simulink model "Ass3_2_2"  (R2018b)
settings: Solver=VariableStepAuto  StartTime=0.0  StopTime=40.0  RelTol=1e-3
values from neighbouring files (symbols this model uses):
  D = [X(3),0,c_0]    [Adaptive3.m]
undefined symbols (not defined in the file or in its folder): sys_m, sys_p
libraries: cstblocks x2
settings Model: Creator=bigfoot  LastModifiedBy=bigfoot

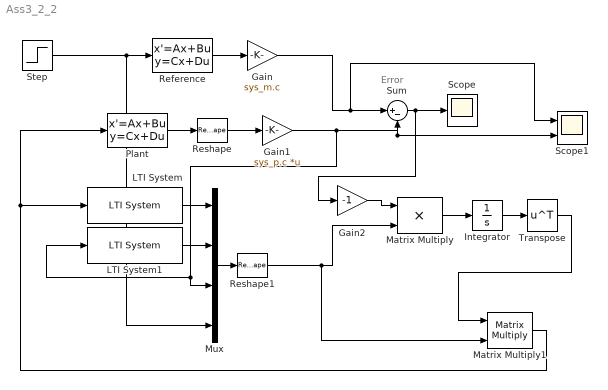
== system Ass3_2_2 ==
  note: Error
  Gain : Gain  Gain=sys_m.c
  Gain1 : Gain  Gain=sys_p.c  Multiplication=Matrix(K*u)
  Gain2 : Gain  Gain=-1
  Integrator : Integrator
  LTI System : cstblocks/LTI System  sys=tf(1,[1 1])  IC=[]
  LTI System1 : cstblocks/LTI System  sys=tf(1,[1 1])  IC=[]
  Matrix Multiply : Product
  Matrix Multiply1 : Product  Multiplication=Matrix(*)
  Mux : Mux
  Plant : StateSpace  A=sys_p.a  B=sys_p.b  C=eye(2)  D=[0;0]  InitialCondition=0
  Reference : StateSpace  A=sys_m.a  B=sys_m.b  C=eye(1)  D=[0]  InitialCondition=0
  Reshape : Reshape  OutputDimensionality=Column vector (2-D)
  Reshape1 : Reshape  OutputDimensionality=Column vector (2-D)
  Scope : Scope
  Scope1 : Scope  NumInputPorts=2
  Step : Step  SampleTime=0
  Sum : Sum  Inputs=|+-
  Transpose : Math  Operator=transpose  SaturateOnIntegerOverflow=on
  wires:
  Sum/1 -> Gain2/1, Scope/1
  Gain/1 -> Scope1/1, Sum/1
  Reference/1 -> Gain/1
  Gain1/1 -> LTI System1/1, Mux/3, Scope1/2, Sum/2
  Plant/1 -> Reshape/1
  Reshape/1 -> Gain1/1
  Step/1 -> Mux/4, Reference/1
  LTI System/1 -> Mux/1
  LTI System1/1 -> Mux/2
  Mux/1 -> Reshape1/1
  Gain2/1 -> Matrix Multiply/1
  Reshape1/1 -> Matrix Multiply1/2, Matrix Multiply/2
  Matrix Multiply/1 -> Integrator/1
  Integrator/1 -> Transpose/1
  Transpose/1 -> Matrix Multiply1/1
  Matrix Multiply1/1 -> LTI System/1, Plant/1
